simulink model "V1_DC_DC"  (R2024b)
settings: Solver=VariableStepAuto  StartTime=0.0  StopTime=10.0  RelTol=1e-3
InitFcn:
  | %% Initialize twist parameters
  | source_V = 0;
  | Ts = 1e-7;
  | 
  | % set the PID parameters
  | Kp = 0.000215;
  | Ti = 7.5175e-5;
  | Td = 0.0;
  | N  = 0.0;
  | Kd = 0.0;
  | 
  | 
  | %Low side parameters
  | twist_low_side_L = 33e-6;
  | twist_low_side_rL = 20e-3; %Modified
  | twist_low_side_C = 47e-6 + 3*4.7e-6;
  | twist_low_side_C_electrolytic = 47e-6;
  | twist_low_side_C_ceramic = 3*4.7e-6;
  | twist_low_side_rC = 700e-3;
  | twist_low_side_rC_ceramic = 0;
  | twist_low_side_adc_R = 150e3+470;
  | 
  | %High side parameters
  | twist_high_side_C = 33e-6*4 + 4.7e-6*12;
  | twist_high_side_rC = 0.1;
  | twist_high_side_adc_R = 1/(1/2e6 + 1/2e6 + 1/(330e3+5.6e3));
  | twist_high_side_feeder_R = 47e3+4.7e3;
  | R_parallel = 1/(1/twist_high_side_adc_R + 1/twist_high_side_feeder_R);
  | tau_VCC = 0.204;
  | tau_desactive = 0.2;
  | twist_R_VCC = (tau_VCC/twist_high_side_C  - twist_high_side_rC)/(1-(tau_VCC/twist_high_side_C - twist_high_side_rC)/R_parallel);
  | 
  | %High side feeder current
  | %load('feeder_current.mat');
  | feeder_VHigh_min = 12;
  | feeder_VHigh_spacing = 6;
  | feeder_duty_min = 0.1;
  | feeder_duty_spacing = 0.4;
  | feeder_Vth_stop = 8.9;
  | feeder_Vth_start = 9.7;
  | feeder_current_upper_rate_limit = 0.386/(20e-3);
  | feeder_current_lower_rate_limit = -500;
  | 
  | %MOSFET parameters
  | twist_FET_Ron = 0.016;
  | twist_FET_Lon = 0;
  | twist_FET_Rd = 0.006;
  | twist_FET_Vf = 0.7;
  | twist_FET_Rs = 1e10;
  | twist_FET_Cs = inf;
  | twist_FET_Clow_Ron = 220e-3;
  | twist_FET_Clow_Rd = 45e-3; %Modified
  | twist_FET_Clow_Vf = 0.7; %Modified
  | 
  | 
  | %Schottky diode parameters
  | twist_shottky_Ron = 0.48; %Modified
  | twist_shottky_Vf = 0.28; %Modified
  | twist_shottky_Rs = 1e10;
  | twist_shottky_Cs = inf;
  | ... (+13 lines)
undefined symbols (not defined in the file): gcbh, sps_rtmsupport, twist_low_side_lC
libraries: spsSeriesRLCBranchLib x14, spsTriangleGeneratorLib x6, spsMosfetLib x6, spsCurrentMeasurementLib x4, spsControlledCurrentSourceLib x3, spsVoltageMeasurementLib x3, spsIdealSwitchLib x2, spsDiodeLib x2, spsDCVoltageSourceLib x1, sps_lib x1
(part 2 of 2)

== system V1_DC_DC/Control system/LEG2 Control/PWM Generator (2-Level)/Sampling/Sync Natural ==
  wt : Inport
  Uref : Inport  Port=2
  Sync_NaturalSampling : Subsystem
  Cr : Outport  VectorParamsAs1DForOutWhenUnconnected=off
  Uref* : Outport  Port=2  VectorParamsAs1DForOutWhenUnconnected=off
  wires:
  Sync_NaturalSampling/2(Cr) -> Cr/1
  Sync_NaturalSampling/1(Uref*) -> Uref*/1
  wt/1 -> Sync_NaturalSampling/2(wt)
  Uref/1 -> Sync_NaturalSampling/1(Uref)

== system V1_DC_DC/Control system/LEG2 Control/PWM Generator (2-Level)/Sampling/Sync Symmetrical ==
  wt : Inport
  Uref : Inport  Port=2
  Sync_SymmetricalSampling : Subsystem
  Cr : Outport  VectorParamsAs1DForOutWhenUnconnected=off
  Uref* : Outport  Port=2  VectorParamsAs1DForOutWhenUnconnected=off
  wires:
  Sync_SymmetricalSampling/2(Cr) -> Cr/1
  Sync_SymmetricalSampling/1(Uref*) -> Uref*/1
  wt/1 -> Sync_SymmetricalSampling/2(wt)
  Uref/1 -> Sync_SymmetricalSampling/1(Uref)

== system V1_DC_DC/Control system/LEG2 Control/PWM Generator (2-Level)/Sampling/Unsync Asymmetrical ==
  wt : Inport
  Uref : Inport  Port=2
  Unsync_AsymmetricalSampling : Subsystem
  term1 : Terminator
  Cr : Outport  VectorParamsAs1DForOutWhenUnconnected=off
  Uref* : Outport  Port=2  VectorParamsAs1DForOutWhenUnconnected=off
  wires:
  wt/1 -> term1/1
  Unsync_AsymmetricalSampling/2(Cr) -> Cr/1
  Unsync_AsymmetricalSampling/1(Uref*) -> Uref*/1
  Uref/1 -> Unsync_AsymmetricalSampling/1(Uref)

== system V1_DC_DC/Control system/LEG2 Control/PWM Generator (2-Level)/Sampling/Unsync Natural ==
  wt : Inport
  Uref : Inport  Port=2
  Unsync_NaturalSampling : Subsystem
  term1 : Terminator
  Cr : Outport  VectorParamsAs1DForOutWhenUnconnected=off
  Uref* : Outport  Port=2  VectorParamsAs1DForOutWhenUnconnected=off
  wires:
  wt/1 -> term1/1
  Unsync_NaturalSampling/2(Cr) -> Cr/1
  Unsync_NaturalSampling/1(Uref*) -> Uref*/1
  Uref/1 -> Unsync_NaturalSampling/1(Uref)

== system V1_DC_DC/Control system/LEG2 Control/PWM Generator (2-Level)/Sampling/Unsync Symmetrical ==
  wt : Inport
  Uref : Inport  Port=2
  Unsync_SymmetricalSampling : Subsystem
  term1 : Terminator
  Cr : Outport  VectorParamsAs1DForOutWhenUnconnected=off
  Uref* : Outport  Port=2  VectorParamsAs1DForOutWhenUnconnected=off
  wires:
  wt/1 -> term1/1
  Unsync_SymmetricalSampling/2(Cr) -> Cr/1
  Unsync_SymmetricalSampling/1(Uref*) -> Uref*/1
  Uref/1 -> Unsync_SymmetricalSampling/1(Uref)

== system V1_DC_DC/Control system/LEG1 Control /PWM Generator (2-Level)/Sampling/Sync Asymmetrical/Sample & Hold ==
  In : Inport
  Enable : EnablePort
  Out : Outport  VectorParamsAs1DForOutWhenUnconnected=off
  wires:
  In/1 -> Out/1

== system V1_DC_DC/Control system/LEG1 Control /PWM Generator (2-Level)/Sampling/Sync Natural/Sync_NaturalSampling ==
  Uref : Inport  Interpolate=off
  wt : Inport  Port=2  Interpolate=off
  Gain1 : Gain  Gain=2/pi  SaturateOnIntegerOverflow=on  OutDataTypeStr=Inherit: Same as input  ParamDataTypeStr=Inherit: Same as input
  Gain4 : Gain  Gain=nF  SaturateOnIntegerOverflow=on  OutDataTypeStr=Inherit: Same as input  ParamDataTypeStr=Inherit: Same as input
  Trigonometric Function : Trigonometry  Operator=asin
  Trigonometric Function3 : Trigonometry
  Uref* : Outport  VectorParamsAs1DForOutWhenUnconnected=off
  Cr : Outport  Port=2  VectorParamsAs1DForOutWhenUnconnected=off
  wires:
  wt/1 -> Gain4/1
  Gain1/1 -> Cr/1
  Trigonometric Function/1 -> Gain1/1
  Trigonometric Function3/1 -> Trigonometric Function/1
  Gain4/1 -> Trigonometric Function3/1
  Uref/1 -> Uref*/1

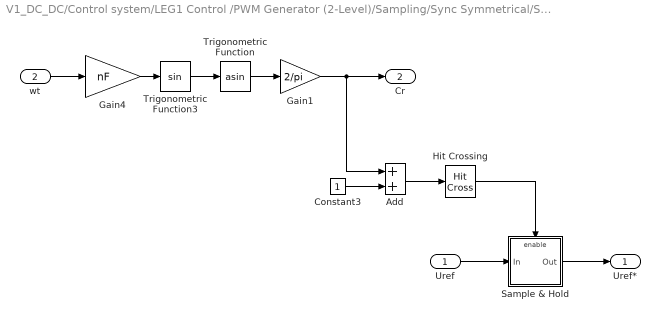
== system V1_DC_DC/Control system/LEG1 Control /PWM Generator (2-Level)/Sampling/Sync Symmetrical/Sync_SymmetricalSampling ==
  Uref : Inport  Interpolate=off
  wt : Inport  Port=2  Interpolate=off
  Add : Sum
  Constant3 : Constant
  Gain1 : Gain  Gain=2/pi  SaturateOnIntegerOverflow=on  OutDataTypeStr=Inherit: Same as input  ParamDataTypeStr=Inherit: Same as input
  Gain4 : Gain  Gain=nF  SaturateOnIntegerOverflow=on  OutDataTypeStr=Inherit: Same as input  ParamDataTypeStr=Inherit: Same as input
  Hit Crossing : HitCross  HitCrossingOffset=1e-9  HitCrossingDirection=falling
  Sample & Hold : Subsystem
  Trigonometric Function : Trigonometry  Operator=asin
  Trigonometric Function3 : Trigonometry
  Uref* : Outport  VectorParamsAs1DForOutWhenUnconnected=off
  Cr : Outport  Port=2  VectorParamsAs1DForOutWhenUnconnected=off
  wires:
  wt/1 -> Gain4/1
  Gain1/1 -> Cr/1, Add/1
  Trigonometric Function/1 -> Gain1/1
  Trigonometric Function3/1 -> Trigonometric Function/1
  Gain4/1 -> Trigonometric Function3/1
  Add/1 -> Hit Crossing/1
  Constant3/1 -> Add/2
  Hit Crossing/1 -> Sample & Hold/Enable
  Uref/1 -> Sample & Hold/1(In)
  Sample & Hold/1(Out) -> Uref*/1

== system V1_DC_DC/Control system/LEG1 Control /PWM Generator (2-Level)/Sampling/Unsync Asymmetrical/Unsync_AsymmetricalSampling ==
  Uref : Inport  Interpolate=off
  Triangle Generator : spsTriangleGeneratorLib/Triangle Generator  Freq=sps.Fc  Phase=sps.Pc  Ts=Ts
  Zero-Order Hold : ZeroOrderHold  SampleTime=sps.SampleTimeZOH_AsymSampling
  Uref* : Outport  VectorParamsAs1DForOutWhenUnconnected=off
  Cr : Outport  Port=2  VectorParamsAs1DForOutWhenUnconnected=off
  wires:
  Triangle Generator/1 -> Cr/1
  Uref/1 -> Zero-Order Hold/1
  Zero-Order Hold/1 -> Uref*/1

== system V1_DC_DC/Control system/LEG1 Control /PWM Generator (2-Level)/Sampling/Unsync Natural/Unsync_NaturalSampling ==
  Uref : Inport  Interpolate=off
  Triangle Generator : spsTriangleGeneratorLib/Triangle Generator  Freq=sps.Fc  Phase=sps.Pc  Ts=Ts
  Uref* : Outport  VectorParamsAs1DForOutWhenUnconnected=off
  Cr : Outport  Port=2  VectorParamsAs1DForOutWhenUnconnected=off
  wires:
  Triangle Generator/1 -> Cr/1
  Uref/1 -> Uref*/1

== system V1_DC_DC/Control system/LEG1 Control /PWM Generator (2-Level)/Sampling/Unsync Symmetrical/Unsync_SymmetricalSampling ==
  Uref : Inport  Interpolate=off
  Triangle Generator : spsTriangleGeneratorLib/Triangle Generator  Freq=sps.Fc  Phase=sps.Pc  Ts=Ts
  Zero-Order Hold : ZeroOrderHold  SampleTime=sps.SampleTimeZOH_SymSampling
  Uref* : Outport  VectorParamsAs1DForOutWhenUnconnected=off
  Cr : Outport  Port=2  VectorParamsAs1DForOutWhenUnconnected=off
  wires:
  Triangle Generator/1 -> Cr/1
  Uref/1 -> Zero-Order Hold/1
  Zero-Order Hold/1 -> Uref*/1

== system V1_DC_DC/Control system/LEG2 Control/PWM Generator (2-Level)/Sampling/Sync Asymmetrical/Sample & Hold ==
  In : Inport
  Enable : EnablePort
  Out : Outport  VectorParamsAs1DForOutWhenUnconnected=off
  wires:
  In/1 -> Out/1

== system V1_DC_DC/Control system/LEG2 Control/PWM Generator (2-Level)/Sampling/Sync Natural/Sync_NaturalSampling ==
  Uref : Inport  Interpolate=off
  wt : Inport  Port=2  Interpolate=off
  Gain1 : Gain  Gain=2/pi  SaturateOnIntegerOverflow=on  OutDataTypeStr=Inherit: Same as input  ParamDataTypeStr=Inherit: Same as input
  Gain4 : Gain  Gain=nF  SaturateOnIntegerOverflow=on  OutDataTypeStr=Inherit: Same as input  ParamDataTypeStr=Inherit: Same as input
  Trigonometric Function : Trigonometry  Operator=asin
  Trigonometric Function3 : Trigonometry
  Uref* : Outport  VectorParamsAs1DForOutWhenUnconnected=off
  Cr : Outport  Port=2  VectorParamsAs1DForOutWhenUnconnected=off
  wires:
  Uref/1 -> Uref*/1
  Gain4/1 -> Trigonometric Function3/1
  Trigonometric Function3/1 -> Trigonometric Function/1
  Trigonometric Function/1 -> Gain1/1
  Gain1/1 -> Cr/1
  wt/1 -> Gain4/1

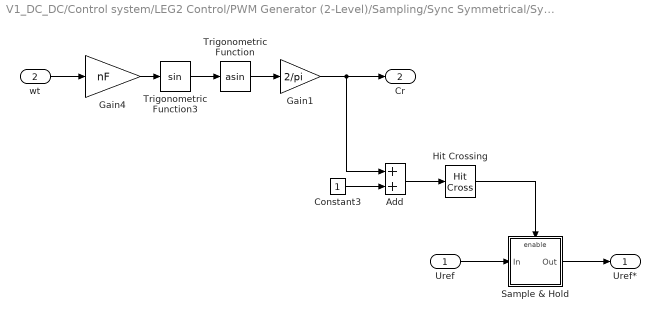
== system V1_DC_DC/Control system/LEG2 Control/PWM Generator (2-Level)/Sampling/Sync Symmetrical/Sync_SymmetricalSampling ==
  Uref : Inport  Interpolate=off
  wt : Inport  Port=2  Interpolate=off
  Add : Sum
  Constant3 : Constant
  Gain1 : Gain  Gain=2/pi  SaturateOnIntegerOverflow=on  OutDataTypeStr=Inherit: Same as input  ParamDataTypeStr=Inherit: Same as input
  Gain4 : Gain  Gain=nF  SaturateOnIntegerOverflow=on  OutDataTypeStr=Inherit: Same as input  ParamDataTypeStr=Inherit: Same as input
  Hit Crossing : HitCross  HitCrossingOffset=1e-9  HitCrossingDirection=falling
  Sample & Hold : Subsystem
  Trigonometric Function : Trigonometry  Operator=asin
  Trigonometric Function3 : Trigonometry
  Uref* : Outport  VectorParamsAs1DForOutWhenUnconnected=off
  Cr : Outport  Port=2  VectorParamsAs1DForOutWhenUnconnected=off
  wires:
  Sample & Hold/1(Out) -> Uref*/1
  Uref/1 -> Sample & Hold/1(In)
  Hit Crossing/1 -> Sample & Hold/Enable
  Constant3/1 -> Add/2
  Add/1 -> Hit Crossing/1
  Gain4/1 -> Trigonometric Function3/1
  Trigonometric Function3/1 -> Trigonometric Function/1
  Trigonometric Function/1 -> Gain1/1
  Gain1/1 -> Add/1, Cr/1
  wt/1 -> Gain4/1

== system V1_DC_DC/Control system/LEG2 Control/PWM Generator (2-Level)/Sampling/Unsync Asymmetrical/Unsync_AsymmetricalSampling ==
  Uref : Inport  Interpolate=off
  Triangle Generator : spsTriangleGeneratorLib/Triangle Generator  Freq=sps.Fc  Phase=sps.Pc  Ts=Ts
  Zero-Order Hold : ZeroOrderHold  SampleTime=sps.SampleTimeZOH_AsymSampling
  Uref* : Outport  VectorParamsAs1DForOutWhenUnconnected=off
  Cr : Outport  Port=2  VectorParamsAs1DForOutWhenUnconnected=off
  wires:
  Zero-Order Hold/1 -> Uref*/1
  Uref/1 -> Zero-Order Hold/1
  Triangle Generator/1 -> Cr/1

== system V1_DC_DC/Control system/LEG2 Control/PWM Generator (2-Level)/Sampling/Unsync Natural/Unsync_NaturalSampling ==
  Uref : Inport  Interpolate=off
  Triangle Generator : spsTriangleGeneratorLib/Triangle Generator  Freq=sps.Fc  Phase=sps.Pc  Ts=Ts
  Uref* : Outport  VectorParamsAs1DForOutWhenUnconnected=off
  Cr : Outport  Port=2  VectorParamsAs1DForOutWhenUnconnected=off
  wires:
  Uref/1 -> Uref*/1
  Triangle Generator/1 -> Cr/1

== system V1_DC_DC/Control system/LEG2 Control/PWM Generator (2-Level)/Sampling/Unsync Symmetrical/Unsync_SymmetricalSampling ==
  Uref : Inport  Interpolate=off
  Triangle Generator : spsTriangleGeneratorLib/Triangle Generator  Freq=sps.Fc  Phase=sps.Pc  Ts=Ts
  Zero-Order Hold : ZeroOrderHold  SampleTime=sps.SampleTimeZOH_SymSampling
  Uref* : Outport  VectorParamsAs1DForOutWhenUnconnected=off
  Cr : Outport  Port=2  VectorParamsAs1DForOutWhenUnconnected=off
  wires:
  Zero-Order Hold/1 -> Uref*/1
  Uref/1 -> Zero-Order Hold/1
  Triangle Generator/1 -> Cr/1

== system V1_DC_DC/Control system/LEG1 Control /PWM Generator (2-Level)/Sampling/Sync Symmetrical/Sync_SymmetricalSampling/Sample & Hold ==
  In : Inport
  Enable : EnablePort
  Out : Outport  VectorParamsAs1DForOutWhenUnconnected=off
  wires:
  In/1 -> Out/1

== system V1_DC_DC/Control system/LEG2 Control/PWM Generator (2-Level)/Sampling/Sync Symmetrical/Sync_SymmetricalSampling/Sample & Hold ==
  In : Inport
  Enable : EnablePort
  Out : Outport  VectorParamsAs1DForOutWhenUnconnected=off
  wires:
  In/1 -> Out/1
